simulink model "CompleteModel_Matfun1"  (R2024b)
settings: Solver=FixedStepAuto  StartTime=0.0  StopTime=10  FixedStep=1  RelTol=1e-3
values from neighbouring files (symbols this model uses):
  Kd = 20    [Model_2811.m]    (also in sat_sim2711.m = diag([0.01, 0.01, 0.01]); satellitemodel2711.m = 1; untitled.m = 1)
  Ki = 0    [Model_2811.m]    (also in sat_sim2711.m = diag([0, 0, 0]); satellitemodel2711.m = 0.1; untitled.m = 10)
  Kp = 50    [Model_2811.m]    (also in sat_sim2711.m = diag([0.05, 0.05, 0.05]); satellitemodel2711.m = 10; untitled.m = 30)
  L_sat = diag([0.06, 0.02, 0.06])    [sat_sim2711.m]
  L_w = 0.05    [sat_sim2711.m]
  omega_desired = [0.1; 0.2; 0.3]    [sat_sim2711.m]
  omega_sat_initial = [0; 0; 0]    [sat_sim2711.m]
settings Model: Creator=LEGION  LastModifiedBy=LEGION

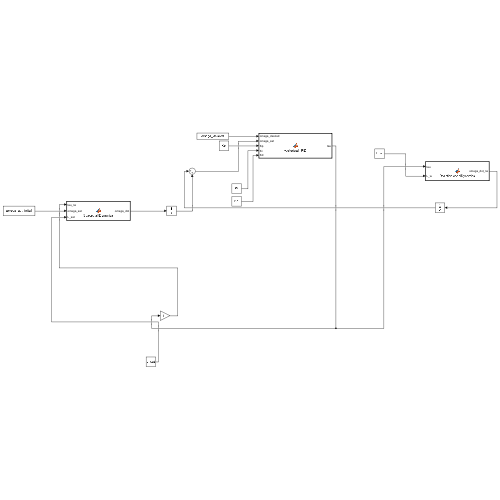
[thumbnail: Simulink's stored preview of the top-level diagram]
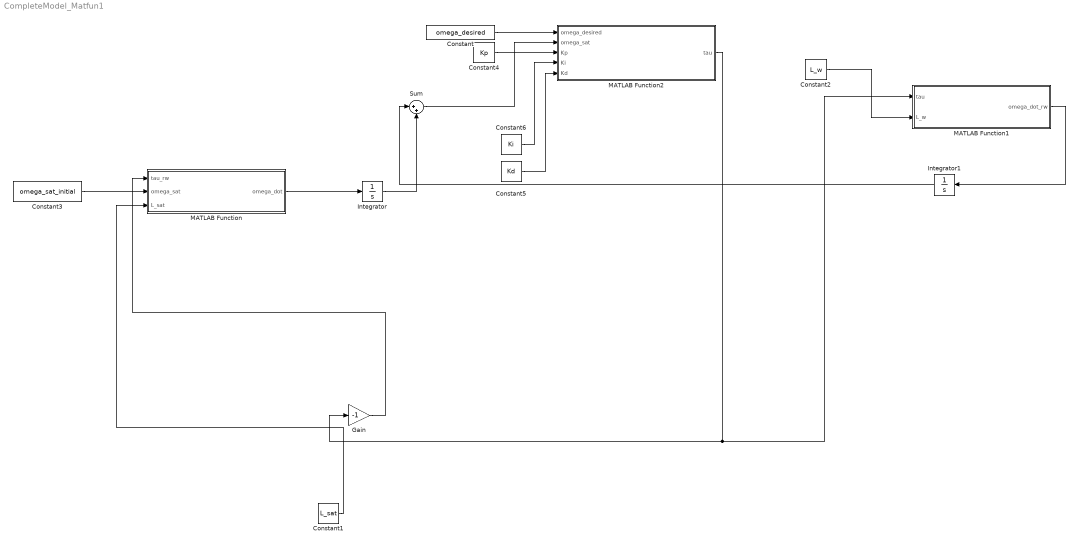
== system CompleteModel_Matfun1 ==
  Constant : Constant  Value=omega_desired
  Constant1 : Constant  Value=L_sat
  Constant2 : Constant  Value=L_w
  Constant3 : Constant  Value=omega_sat_initial
  Constant4 : Constant  Value=Kp
  Constant5 : Constant  Value=Kd
  Constant6 : Constant  Value=Ki
  Gain : Gain  Gain=-1
  Integrator : Integrator
  Integrator1 : Integrator
  MATLAB Function : MATLAB Function  TreatAsAtomicUnit=on
  MATLAB Function1 : MATLAB Function  TreatAsAtomicUnit=on
  MATLAB Function2 : MATLAB Function  TreatAsAtomicUnit=on
  Sum : Sum  Inputs=|++
  wires:
  Constant1/1 -> MATLAB Function/3(L_sat)
  Constant2/1 -> MATLAB Function1/2(L_w)
  Constant3/1 -> MATLAB Function/2(omega_sat)
  Gain/1 -> MATLAB Function/1(tau_rw)
  Constant5/1 -> MATLAB Function2/5(Kd)
  Constant4/1 -> MATLAB Function2/3(Kp)
  Constant6/1 -> MATLAB Function2/4(Ki)
  MATLAB Function/1(omega_dot) -> Integrator/1
  Integrator/1 -> Sum/2
  MATLAB Function1/1(omega_dot_rw) -> Integrator1/1
  Integrator1/1 -> Sum/1
  Sum/1 -> MATLAB Function2/2(omega_sat)
  Constant/1 -> MATLAB Function2/1(omega_desired)
  MATLAB Function2/1(tau) -> Gain/1, MATLAB Function1/1(tau)

== matlab function CompleteModel_Matfun1/MATLAB Function1 ==
  data: tau input; omega_dot_rw output; L_w input
function omega_dot_rw =  ReactionwheelDynamics( tau, L_w)

tau_rw = -tau; % Equal and opposite to spacecraft torque
omega_dot_rw = tau / L_w;

== matlab function CompleteModel_Matfun1/MATLAB Function ==
  data: tau_rw input; omega_dot output; omega_sat input; L_sat input
function omega_dot =  SpacecraftDynamics( tau_rw,omega_sat, L_sat)

omega_dot = inv(L_sat) * (tau_rw - cross(omega_sat, L_sat*omega_sat));

== matlab function CompleteModel_Matfun1/MATLAB Function2 ==
  data: omega_desired input; tau output; omega_sat input; Kp input; Ki input; Kd input
function tau = vectorized_PID(omega_desired, omega_sat, Kp, Ki, Kd)
    % Error calculation
    error = omega_desired - omega_sat;

    % Proportional control
    proportional = Kp .* error;

    % Integral control (optional, for simplicity assume you sum the error over time)
    integral = Ki .* cumsum(error);

    % Derivative control (change in omega_sat, assuming omega_sat is 3x1 vector)
    derivative = Kd .* diff([omega_sat(1, :); omega_sat], 1, 1);  % Ensures it computes over the correct axis

    % Combined output
    tau = proportional + integral + derivative;
end
